simulink model "mancal_v2"  (R2013a)
settings: Solver=ode45  StartTime=0.0  StopTime=3  RelTol=1e-5
values from neighbouring files (symbols this model uses):
  dA = [1.435e2 3.335e-2]    [parametriza.m]    (also in parametrizaMancal.m)
  E = 3e9    (= 3000000000)    [parametriza.m]    (also in parametrizaMancal.m)
  gb = 0.4e-3    (= 0.0004)    [main.m]    (also in parametriza.m = 0.0003; parametrizaMancal.m)
  gi = 0.6e-3    (= 0.0006)    [main.m]    (also in parametriza.m = 0.0007; parametrizaMancal.m)
  Hb = 8e-3    (= 0.008)    [parametriza.m]    (also in parametrizaMancal.m)
  Kb = 46.53E3    (= 46530)    [main.m]    (also in parametriza.m = 58; parametrizaMancal.m = E*Hb*Ab/Lb)
  Ke = [3.8e-9 2.86e-3]    [parametrizaMancal.m]
  Km = 540e3    (= 540000)    [parametrizaMancal.m]
  L = [-57.6135 0.0908]    [main.m]    (also in parametriza.m = tf(Kb,[L2 R]); parametrizaMancal.m)
  Lb = 5.3e-3    (= 0.0053)    [parametriza.m]    (also in parametrizaMancal.m)
  m = 4.7e-5*7.86e3    (= 0.36942)    [main.m]    (also in parametriza.m = 0.375; parametrizaMancal.m)
  N = 300    [main.m]    (also in parametriza.m; parametrizaMancal.m)
  R = 4    [main.m]    (also in parametriza.m = 6.3; parametrizaMancal.m)
  Vmax = 30    [parametriza.m]    (also in parametrizaMancal.m)
undefined symbols (not defined in the file or in its folder): C
libraries: simulink x1, dspmathops x1
settings Model: Creator=leo  LastModifiedBy=rafa
settings OptimizationCC: AccelVerboseBuild=on
settings DebuggingCC: SolverPrmCheckMsg=none
settings ModelReferenceCC: UpdateModelReferenceTargets=IfOutOfDate
settings SFSimCC: SFSimEcho=off

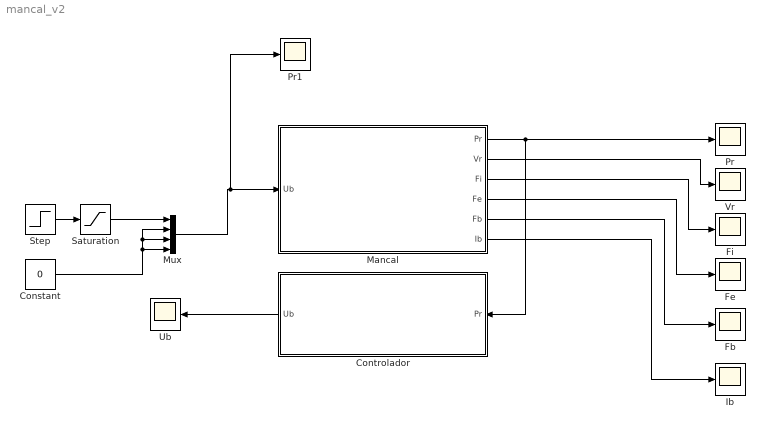
== system mancal_v2 ==
  Constant : Constant  Value=0
  Controlador : Subsystem
  Fb : Scope
      settings: YMin=-200000  YMax=200000  SaveName=scope_fb
  Fe : Scope
      settings: YMin=-500  YMax=25  SaveName=scope_fe
  Fi : Scope
      settings: YMin=0  YMax=450  SaveName=ScopeData3
  Ib : Scope
      settings: YMin=0  YMax=7.5  SaveName=scope_ib
  Mancal : Subsystem
  Mux : Mux
  Pr : Scope
      settings: TimeRange=0.03612231404958678  YMin=7.472330934646299e-05  YMax=0.0004236018179522787  SaveName=scope_pr
  Pr1 : Scope
      settings: TimeRange=3  YMin=5.55112e-17  YMax=2.2  SaveName=scope_vb
  Saturation : Saturate  UpperLimit=30  LowerLimit=0
  Step : Step  After=10  SampleTime=0
  Ub : Scope
      settings: TimeRange=0.1  YMin=0  YMax=10  SaveName=ScopeData10
  Vr : Scope
      settings: YMin=-45  YMax=45
  wires:
  Mancal/1(Pr) -> Controlador/1(Pr), Pr/1
  Mancal/2(Vr) -> Vr/1
  Mancal/4(Fe) -> Fe/1
  Mancal/3(Fi) -> Fi/1
  Mancal/6(Ib) -> Ib/1
  Mancal/5(Fb) -> Fb/1
  Controlador/1(Ub) -> Ub/1
  Step/1 -> Saturation/1
  Constant/1 -> Mux/2, Mux/3, Mux/4
  Mux/1 -> Pr1/1, Mancal/1(Ub)
  Saturation/1 -> Mux/1

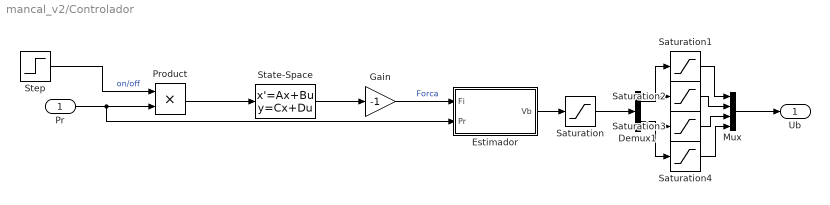
== system mancal_v2/Controlador ==
  Pr : Inport
  Demux1 : Demux  Outputs=2
  Estimador : Subsystem
  Gain : Gain  Gain=-1
  Mux : Mux
  Product : Product
  Saturation : Saturate  UpperLimit=Vmax  LowerLimit=-Vmax
  Saturation1 : Saturate  UpperLimit=Inf  LowerLimit=0
  Saturation2 : Saturate  UpperLimit=0  LowerLimit=-Inf
  Saturation3 : Saturate  UpperLimit=Inf  LowerLimit=0
  Saturation4 : Saturate  UpperLimit=0  LowerLimit=-Inf
  State-Space : StateSpace  A=ss([C 1; 1 C]).A  B=ss([C 1; 1 C]).B  C=ss([C 1; 1 C]).C  D=ss([C 1; 1 C]).D
  Step : Step  SampleTime=0
  Ub : Outport
  wires:
  Mux/1 -> Ub/1
  Saturation/1 -> Demux1/1
  Saturation4/1 -> Mux/4
  Saturation3/1 -> Mux/3
  Saturation2/1 -> Mux/2
  Saturation1/1 -> Mux/1
  Demux1/2 -> Saturation3/1, Saturation4/1
  Demux1/1 -> Saturation2/1, Saturation1/1
  Gain/1 -> Estimador/1(Fi)  "Forca"
  Estimador/1(Vb) -> Saturation/1
  State-Space/1 -> Gain/1
  Product/1 -> State-Space/1
  Pr/1 -> Product/2, Estimador/2(Pr)
  Step/1 -> Product/1  "on/off"

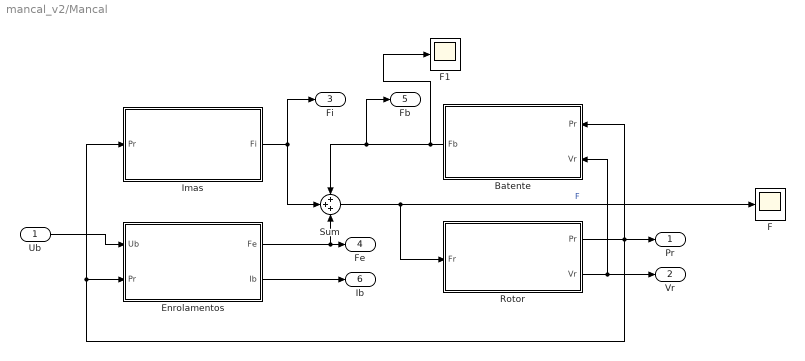
== system mancal_v2/Mancal ==
  Ub : Inport
  Batente : Subsystem
  Enrolamentos : Subsystem
  F : Scope
      settings: TimeRange=1  YMin=-200000  YMax=200000  SaveName=ScopeData13
  F1 : Scope
      settings: TimeRange=1  YMin=-200000  YMax=200000  SaveName=ScopeData14
  Imas : Subsystem
  Rotor : Subsystem
  Sum : Sum  Inputs=+++
  Pr : Outport
  Vr : Outport  Port=2
  Fi : Outport  Port=3
  Fe : Outport  Port=4
  Fb : Outport  Port=5
  Ib : Outport  Port=6
  wires:
  Sum/1 -> Rotor/1(Fr), F/1  "F"
  Ub/1 -> Enrolamentos/1(Ub)
  Enrolamentos/1(Fe) -> Sum/3, Fe/1
  Enrolamentos/2(Ib) -> Ib/1
  Batente/1(Fb) -> F1/1, Sum/1, Fb/1
  Rotor/1(Pr) -> Batente/1(Pr), Pr/1, Imas/1(Pr), Enrolamentos/2(Pr)
  Rotor/2(Vr) -> Batente/2(Vr), Vr/1
  Imas/1(Fi) -> Sum/2, Fi/1

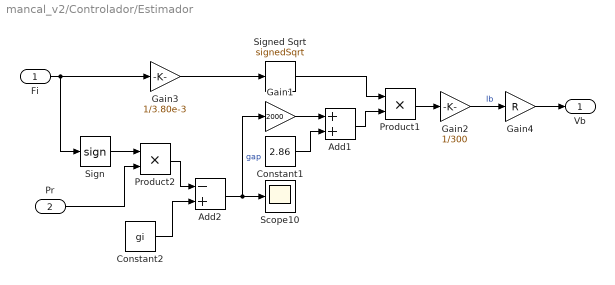
== system mancal_v2/Controlador/Estimador ==
  Fi : Inport
  Pr : Inport  Port=2
  Add1 : Sum
  Add2 : Sum  Inputs=-+
  Constant1 : Constant  Value=2.86
  Constant2 : Constant  Value=gi
  Gain1 : Gain  Gain=2000
  Gain2 : Gain  Gain=1/300
  Gain3 : Gain  Gain=1/3.80e-3
  Gain4 : Gain  Gain=R
  Product1 : Product
  Product2 : Product
  Scope10 : Scope
      settings: TimeRange=2.85171102661597  YMin=0.0002  YMax=0.001  SaveName=ScopeData11
  Sign : Signum
  Signed Sqrt : Sqrt  Operator=signedSqrt  SaturateOnIntegerOverflow=on
  Vb : Outport
  wires:
  Constant2/1 -> Add2/2
  Product2/1 -> Add2/1
  Pr/1 -> Product2/2
  Sign/1 -> Product2/1
  Gain4/1 -> Vb/1
  Product1/1 -> Gain2/1
  Add2/1 -> Scope10/1, Gain1/1  "gap"
  Constant1/1 -> Add1/2
  Signed Sqrt/1 -> Product1/1
  Gain2/1 -> Gain4/1  "Ib"
  Gain3/1 -> Signed Sqrt/1
  Gain1/1 -> Add1/1
  Fi/1 -> Sign/1, Gain3/1
  Add1/1 -> Product1/2

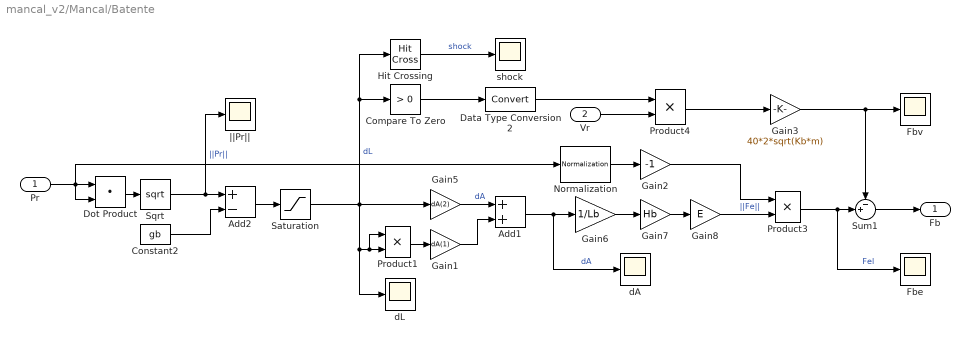
== system mancal_v2/Mancal/Batente ==
  Pr : Inport
  Vr : Inport  Port=2
  Add1 : Sum
  Add2 : Sum  Inputs=+-
  Compare To Zero : simulink/Logic and Bit Operations/Compare To Zero  relop=>  OutDataTypeStr=boolean
  Constant2 : Constant  Value=gb
  Data Type Conversion2 : DataTypeConversion
  Dot Product : DotProduct  InputSameDT=on  OutDataTypeStr=Inherit: Inherit via internal rule
  Fbe : Scope
      settings: TimeRange=0.0002829354553492485  YMin=-100000  YMax=100000  SaveName=ScopeData15
  Fbv : Scope
      settings: TimeRange=0.1  YMin=-225000  YMax=225000  SaveName=ScopeData8
  Gain1 : Gain  Gain=dA(1)
  Gain2 : Gain  Gain=-1
  Gain3 : Gain  Gain=40*2*sqrt(Kb*m)
  Gain5 : Gain  Gain=dA(2)
  Gain6 : Gain  Gain=1/Lb
  Gain7 : Gain  Gain=Hb
  Gain8 : Gain  Gain=E
  Hit Crossing : HitCross  HitCrossingDirection=rising
  Normalization : dspmathops/Normalization  NormType=2-norm  Bias=1e-10  NormOver=Each column  ColComp=on  Dimension=1  outputDataTypeStr=Inherit: Same as product output  outputLastDataTypeStr=Inherit: Same as product output  outputMin=[]  outputMax=[]  accumDataTypeStr=Inherit: Same as product output  accumLastDataTypeStr=Inherit: Same as product output  roundingMode=Floor  overflowMode=off
  Product1 : Product
  Product3 : Product
  Product4 : Product
  Saturation : Saturate  UpperLimit=Inf  LowerLimit=0
  Sqrt : Sqrt  SaturateOnIntegerOverflow=on
  Sum1 : Sum  Inputs=-+|
  dA : Scope
      settings: TimeRange=0.0002829354553492485  YMin=3.91545e-05  YMax=3.9158e-05  SaveName=ScopeData4
  dL : Scope
      settings: TimeRange=0.1  YMin=1.4215e-06  YMax=1.4315e-06  SaveName=ScopeData7
  shock : Scope
      settings: TimeRange=0.0002829354553492485  YMin=5.54637e-16  YMax=5.54639e-16  SaveName=ScopeData19
  ||Pr|| : Scope
      settings: TimeRange=0.0002829354553492485  YMin=-2.75  YMax=0  SaveName=ScopeData18
  Fb : Outport
  wires:
  Dot Product/1 -> Sqrt/1
  Gain8/1 -> Product3/2  "||Fe||"
  Compare To Zero/1 -> Data Type Conversion2/1
  Saturation/1 -> dL/1, Product1/1, Product1/2, Hit Crossing/1, Compare To Zero/1, Gain5/1  "dL"
  Add2/1 -> Saturation/1
  Sqrt/1 -> ||Pr||/1, Add2/1  "||Pr||"
  Constant2/1 -> Add2/2
  Gain6/1 -> Gain7/1
  Gain7/1 -> Gain8/1
  Product4/1 -> Gain3/1
  Product3/1 -> Sum1/2, Fbe/1  "Fel"
  Sum1/1 -> Fb/1
  Data Type Conversion2/1 -> Product4/1
  Product1/1 -> Gain1/1
  Gain5/1 -> Add1/1  "dA"
  Add1/1 -> dA/1, Gain6/1  "dA"
  Gain3/1 -> Fbv/1, Sum1/1
  Vr/1 -> Product4/2
  Normalization/1 -> Gain2/1
  Pr/1 -> Normalization/1, Dot Product/2, Dot Product/1
  Gain2/1 -> Product3/1
  Gain1/1 -> Add1/2
  Hit Crossing/1 -> shock/1  "shock"

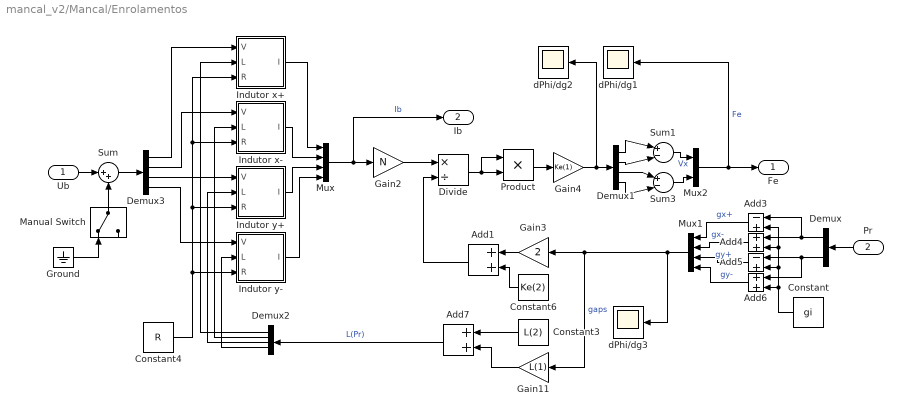
== system mancal_v2/Mancal/Enrolamentos ==
  Ub : Inport
  Pr : Inport  Port=2
  Add{1,4,6..7} (4 alike) : Sum
  Add3 : Sum  Inputs=-+
  Add5 : Sum  Inputs=-+
  Constant : Constant  Value=gi
  Constant3 : Constant  Value=L(2)
  Constant4 : Constant  Value=R
  Constant6 : Constant  Value=Ke(2)
  Demux : Demux  Outputs=2
  Demux1 : Demux
  Demux2 : Demux
  Demux3 : Demux
  Divide : Product  Inputs=*/
  Gain11 : Gain  Gain=L(1)
  Gain2 : Gain  Gain=N
  Gain3 : Gain  Gain=2
  Gain4 : Gain  Gain=Ke(1)
  Ground : Ground
  Indutor x+ : Subsystem
  Indutor x- : Subsystem
  Indutor y+ : Subsystem
  Indutor y- : Subsystem
  Manual Switch : ManualSwitch
  Mux : Mux
  Mux1 : Mux
  Mux2 : Mux  Inputs=2
  Product : Product
  Sum : Sum  Inputs=|++
  Sum1 : Sum  Inputs=|+-|
  Sum3 : Sum  Inputs=|+-|
  dPhi/dg1 : Scope
      settings: TimeRange=0.0002829354553492485  YMin=-100000  YMax=100000
  dPhi/dg2 : Scope
      settings: TimeRange=0.0002829354553492485  YMin=0  YMax=1900  SaveName=ScopeData20
  dPhi/dg3 : Scope
      settings: TimeRange=0.0002829354553492485  YMin=0  YMax=1900  SaveName=ScopeData12
  Fe : Outport
  Ib : Outport  Port=2
  wires:
  Add1/1 -> Divide/2
  Gain2/1 -> Divide/1
  Product/1 -> Gain4/1
  Gain3/1 -> Add1/1
  Constant/1 -> Add5/2, Add4/2, Add3/2, Add6/2
  Constant6/1 -> Add1/2
  Divide/1 -> Product/2, Product/1
  Mux/1 -> Ib/1, Gain2/1  "Ib"
  Demux1/2 -> Sum1/2
  Demux3/3 -> Indutor y+/1(V)
  Demux3/2 -> Indutor x-/1(V)
  Indutor x-/1(I) -> Mux/2
  Indutor y+/1(I) -> Mux/3
  Indutor y-/1(I) -> Mux/4
  Gain4/1 -> dPhi/dg2/1, Demux1/1
  Mux2/1 -> dPhi/dg1/1, Fe/1  "Fe"
  Sum3/1 -> Mux2/2
  Sum1/1 -> Mux2/1  "Vx"
  Demux1/4 -> Sum3/2
  Demux1/1 -> Sum1/1
  Demux1/3 -> Sum3/1
  Add3/1 -> Mux1/1  "gx+"
  Add4/1 -> Mux1/2  "gx-"
  Add5/1 -> Mux1/3  "gy+"
  Add6/1 -> Mux1/4  "gy-"
  Mux1/1 -> dPhi/dg3/1, Gain3/1, Gain11/1  "gaps"
  Demux/1 -> Add4/1, Add3/1
  Demux/2 -> Add5/1, Add6/1
  Demux3/4 -> Indutor y-/1(V)
  Add7/1 -> Demux2/1  "L(Pr)"
  Constant4/1 -> Indutor x+/3(R), Indutor x-/3(R), Indutor y+/3(R), Indutor y-/3(R)
  Constant3/1 -> Add7/1
  Gain11/1 -> Add7/2
  Demux2/2 -> Indutor x-/2(L)
  Demux2/3 -> Indutor y+/2(L)
  Demux2/4 -> Indutor y-/2(L)
  Indutor x+/1(I) -> Mux/1
  Demux2/1 -> Indutor x+/2(L)
  Pr/1 -> Demux/1
  Demux3/1 -> Indutor x+/1(V)
  Ub/1 -> Sum/1
  Sum/1 -> Demux3/1
  Manual Switch/1 -> Sum/2
  Ground/1 -> Manual Switch/1

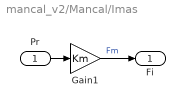
== system mancal_v2/Mancal/Imas ==
  Pr : Inport
  Gain1 : Gain  Gain=Km
  Fi : Outport
  wires:
  Pr/1 -> Gain1/1
  Gain1/1 -> Fi/1  "Fm"

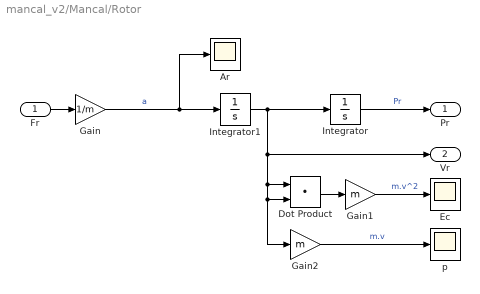
== system mancal_v2/Mancal/Rotor ==
  Fr : Inport
  Ar : Scope
      settings: TimeRange=1  YMin=-200000  YMax=200000  SaveName=ScopeData9
  Dot Product : DotProduct  InputSameDT=on  OutDataTypeStr=Inherit: Inherit via internal rule
  Ec : Scope
      settings: TimeRange=0.25  YMin=0  YMax=0.09  SaveName=ScopeData16
  Gain : Gain  Gain=1/m
  Gain1 : Gain  Gain=m
  Gain2 : Gain  Gain=m
  Integrator : Integrator  InitialCondition=[.001 .002]*1e-3  UpperSaturationLimit=Inf  LowerSaturationLimit=-Inf
  Integrator1 : Integrator
  p : Scope
      settings: TimeRange=1  YMin=-200000  YMax=200000  SaveName=ScopeData17
  Pr : Outport
  Vr : Outport  Port=2
  wires:
  Fr/1 -> Gain/1
  Integrator/1 -> Pr/1  "Pr"
  Gain/1 -> Ar/1, Integrator1/1  "a"
  Dot Product/1 -> Gain1/1
  Integrator1/1 -> Dot Product/1, Gain2/1, Dot Product/2, Vr/1, Integrator/1
  Gain2/1 -> p/1  "m.v"
  Gain1/1 -> Ec/1  "m.v^2"

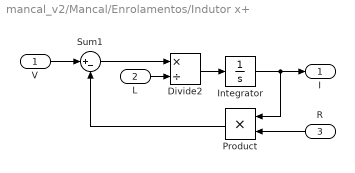
== system mancal_v2/Mancal/Enrolamentos/Indutor x+ ==
  V : Inport
  L : Inport  Port=2
  R : Inport  Port=3
  Divide2 : Product  Inputs=*/
  Integrator : Integrator
  Product : Product
  Sum1 : Sum  Inputs=|+-
  I : Outport
  wires:
  Divide2/1 -> Integrator/1
  Sum1/1 -> Divide2/1
  Integrator/1 -> Product/1, I/1
  Product/1 -> Sum1/2
  L/1 -> Divide2/2
  V/1 -> Sum1/1
  R/1 -> Product/2

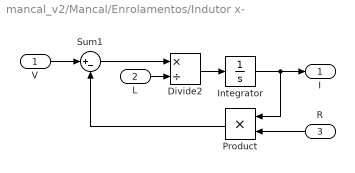
== system mancal_v2/Mancal/Enrolamentos/Indutor x- ==
  V : Inport
  L : Inport  Port=2
  R : Inport  Port=3
  Divide2 : Product  Inputs=*/
  Integrator : Integrator
  Product : Product
  Sum1 : Sum  Inputs=|+-
  I : Outport
  wires:
  R/1 -> Product/2
  V/1 -> Sum1/1
  L/1 -> Divide2/2
  Product/1 -> Sum1/2
  Integrator/1 -> I/1, Product/1
  Sum1/1 -> Divide2/1
  Divide2/1 -> Integrator/1

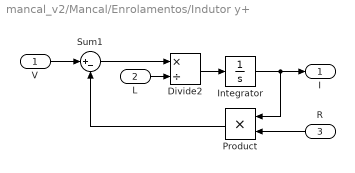
== system mancal_v2/Mancal/Enrolamentos/Indutor y+ ==
  V : Inport
  L : Inport  Port=2
  R : Inport  Port=3
  Divide2 : Product  Inputs=*/
  Integrator : Integrator
  Product : Product
  Sum1 : Sum  Inputs=|+-
  I : Outport
  wires:
  R/1 -> Product/2
  V/1 -> Sum1/1
  L/1 -> Divide2/2
  Product/1 -> Sum1/2
  Integrator/1 -> I/1, Product/1
  Sum1/1 -> Divide2/1
  Divide2/1 -> Integrator/1

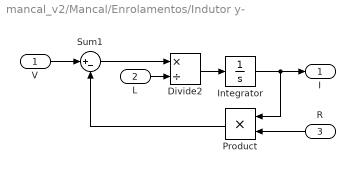
== system mancal_v2/Mancal/Enrolamentos/Indutor y- ==
  V : Inport
  L : Inport  Port=2
  R : Inport  Port=3
  Divide2 : Product  Inputs=*/
  Integrator : Integrator
  Product : Product
  Sum1 : Sum  Inputs=|+-
  I : Outport
  wires:
  R/1 -> Product/2
  V/1 -> Sum1/1
  L/1 -> Divide2/2
  Product/1 -> Sum1/2
  Integrator/1 -> I/1, Product/1
  Sum1/1 -> Divide2/1
  Divide2/1 -> Integrator/1
